simulink model "soc_learn_fpga"  (R2025b)
settings: Solver=FixedStepDiscrete  StartTime=0.0  StopTime=1e-6  FixedStep=8e-09  RelTol=1e-3  EnableMultiTasking=on
model workspace (MAT data in the model file):
  socvcb = containers.Map
  socvcb.serialization.keys = {155.255737305}
  socvcb.serialization.values : function handle (value not decoded)
  socvcb.serialization.uniformity = 0
  socvcb.serialization.keyType = 'double'
  socvcb.serialization.valueType = 'any'
undefined symbols (not defined in the file): AXI4, Stream
libraries: socmemlib x1, hwlogicconnlib x1
settings Model: Creator=kimsteph  LastModifiedBy=kimsteph
settings SolverCC: PositivePriorityOrder=on
settings OptimizationCC: DefaultParameterBehavior=Inlined  EnhancedBackFolding=on  PassReuseOutputArgsAs=Individual arguments  ZeroExternalMemoryAtStartup=off  ZeroInternalMemoryAtStartup=off  MaxStackSize=64  OptimizeBlockOrder=speed  DifferentSizesBufferReuse=on  OptimizationCustomize=off  EfficientTunableParamExpr=on
settings DebuggingCC: ParameterTunabilityLossMsg=error
settings HardwareCC: ProdBitPerLong=64.0  ProdLargestAtomicInteger=LongLong  ProdLargestAtomicFloat=Double  ProdLongLongMode=on  ProdHWDeviceType=ARM Compatible->ARM Cortex-A (64-bit)  HardwareBoardFeatureSet=SoCBlockset
settings ModelReferenceCC: ModelReferenceNumInstancesAllowed=Single
settings SFSimCC: MATLABDynamicMemAlloc=off
settings RTWCC: SystemTargetFile=ert.tlc  HardwareBoard=Xilinx Zynq UltraScale+ RFSoC ZCU111 Evaluation Kit  TLCOptions="-aInlineSetEventsForThisBaseRateFcn=TLC_FALSE -aSuppressMultiTaskScheduler=TLC_FALSE  -aRateBasedStepFcn=0"  TemplateMakefile=ert_default_tmf  Toolchain=Linaro AArch64 Linux v6.3.1  Description=Embedded Coder
settings CodeAppCC: ForceParamTrailComments=on  IgnoreCustomStorageClasses=off  OperatorAnnotations=on  SimulinkDataObjDesc=on  SFDataObjDesc=on  InsertBlockDesc=on
settings ERTTargetCC: SubcomponentCodeInterfacePackaging=Nonreusable function

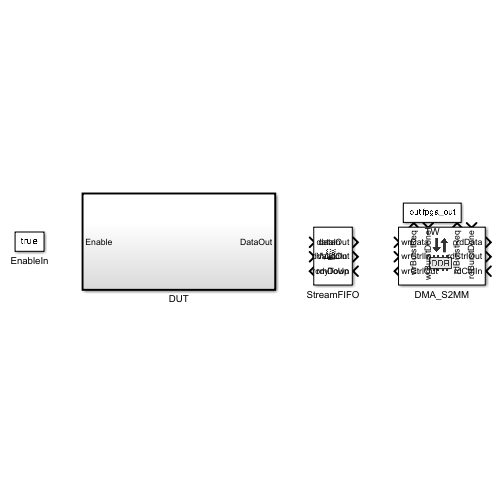
[thumbnail: Simulink's stored preview of the top-level diagram]
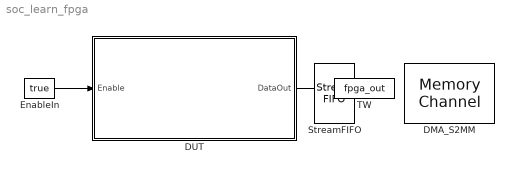
== system soc_learn_fpga ==
  DMA_S2MM : socmemlib/Memory Channel  InstantiateOnLoad=on  EnableMemSim=on  ChannelType=AXI4-Stream FIFO  MRBufferSize=4096  MRNumBuffers=8  BurstLengthWriterChIf=256  BurstLengthReaderChIf=256  UseValuesFromTargetHardwareResources=off  ReaderWriterUseSameValues=on  FIFODepthWriter=8  FIFODepthReader=8  FIFOAFullDepthWriter=6  FIFOAFullDepthReader=6  ICClockFrequencyWriter=100  ICClockFrequencyReader=100  ICDataWidthWriter=32  ICDataWidthReader=32  ChDimensionsWriterChIf=1024  ChTypeWriterChIf=uint32  ChFrameSampleTimeWriterChIf=1  ChBitPackedWriterChIf=off  OutSigSpecMatchesInSigSpec=on  ChDimensionsReaderChIf=1024  ChTypeWithInhReaderChIf=uint32  ChFrameSampleTimeReaderChIf=1  ChBitPackedReaderChIf=off  ChSampleTimeOffsetReaderChIf=on  InsertInactivePixelClocksReaderChIf=off  FrameSizeReaderChIf=160x120p  ProtocolWriter=AXI4-Stream  ProtocolReader=AXI4-Stream  ChTypeReaderChIf=uint32  LastTargetBoard=Xilinx Zynq UltraScale+ RFSoC ZCU111 Evaluation Kit  Beta2Compatible=off  MRRegionSize=32768  DiagnosticLevel=No debug  MRBaseAddress=hex2dec('00010000')  UseTargetGlobalValues=off  InterruptHandlingTimeWriterChIf=10e-6  BufferEventIDWriterChIf=NOT_USED  BufferLengthReaderChIf=NOT_USED  InterruptHandlingTimeReaderChIf=10e-6  BufferEventIDReaderChIf=NOT_USED
  DUT : Subsystem  TreatAsAtomicUnit=on
  EnableIn : Constant  Value=true  OutDataTypeStr=boolean
  StreamFIFO : hwlogicconnlib/Stream FIFO  FIFO_DEPTH=16  AFULL_THRESH=8
  TW : ToWorkspace  VariableName=fpga_out  SaveFormat=Timeseries  SampleTime=-1
  wires:
  EnableIn/1 -> DUT/1(Enable)
  DUT/1(DataOut) -> TW/1

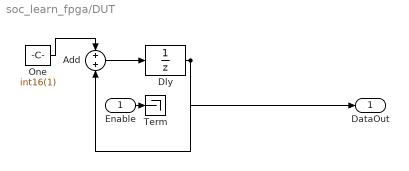
== system soc_learn_fpga/DUT ==
  Enable : Inport  OutDataTypeStr=boolean
  Add : Sum  OutDataTypeStr=int16
  Dly : UnitDelay  SampleTime=8e-09  HasFrameUpgradeWarning=on
  One : Constant  Value=int16(1)  OutDataTypeStr=int16
  Term : Terminator
  DataOut : Outport
  wires:
  One/1 -> Add/1
  Dly/1 -> Add/2, DataOut/1
  Add/1 -> Dly/1
  Enable/1 -> Term/1
